simulink model "scdcascade_breach"  (R2020a)
settings: Solver=ode45  StartTime=0.0  StopTime=tspan(end)  RelTol=1e-3  EnableMultiTasking=on
PreLoadFcn:
  | Kp2 = 1.4817;
  | Ki2 = 4.7555;
  | Kp1 = 0.1575;
  | Ki1 = 0.042;
model workspace (MAT data in the model file):
  C1 = pidstd
  C1.IOSize_ = [1 1]
  C1.Data_ = ltipack.piddataS
  C1.Data_.Delay.Input = 0
  C1.Data_.Delay.Output = 0
  C1.Data_.Delay.IO = 0
  C1.Data_.Ts = 0
  C1.Data_.Kp = 0.1
  C1.Data_.Ti = 1
  C1.Data_.Td = 0
  C1.Data_.N = Inf
  C2 = pidstd
  C2.IOSize_ = [1 1]
  C2.Data_ = ltipack.piddataS
  C2.Data_.Delay.Input = 0
  C2.Data_.Delay.Output = 0
  C2.Data_.Delay.IO = 0
  C2.Data_.Ts = 0
  C2.Data_.Kp = 0.1
  C2.Data_.Ti = 1
  C2.Data_.Td = 0
  C2.Data_.N = Inf
  G1 = zpk
  G1.IOSize_ = [1 1]
  G1.Data_ = ltipack.zpkdata
  G1.Data_.z = {[]}
  G1.Data_.p = {[-1; -1; -1]}
  G1.Data_.k = 10
  G1.Data_.Delay.Input = 0
  G1.Data_.Delay.Output = 0
  G1.Data_.Delay.IO = 0
  G1.Data_.Ts = 0
  G2 = zpk
  G2.IOSize_ = [1 1]
  G2.Data_ = ltipack.zpkdata
  G2.Data_.z = {[]}
  G2.Data_.p = {-2}
  G2.Data_.k = 3
  G2.Data_.Delay.Input = 0
  G2.Data_.Delay.Output = 0
  G2.Data_.Delay.IO = 0
  G2.Data_.Ts = 0
libraries: cstblocks x2, simulink x1
settings Model: FPTRunName=Active  Creator=The MathWorks, Inc.  LastModifiedBy=nikhil
settings DataIOCC: ExternalInput=[t__, u__]  LoadExternalInput=on  SaveFormat=StructureWithTime
settings OptimizationCC: ExpressionDepthLimit=2147483647  LifeSpan=inf
settings DebuggingCC: UnderspecifiedInitializationDetection=Classic  MergeDetectMultiDrivingBlocksExec=none  SolverPrmCheckMsg=warning  FcnCallInpInsideContextMsg=warning  StateNameClashWarn=warning  SFUnexpectedBacktrackingDiag=warning  SFNoUnconditionalDefaultTransitionDiag=warning  SFExecutionAtInitializationDiag=none  ArithmeticOperatorsInVariantConditions=warning
settings HardwareCC: ProdBitPerPointer=32  ProdBitPerSizeT=32  ProdBitPerPtrDiffT=32  ProdLargestAtomicFloat=None  ProdIntDivRoundTo=Undefined  ProdEndianess=Unspecified  ProdWordSize=32  ProdHWDeviceType=32-bit Generic
settings ModelReferenceCC: PropagateSignalLabelsOutOfModel=off
settings SFSimCC: SimUseLocalCustomCode=off  CustomCodeUndefinedFunction=UseInterfaceOnly
settings RTWCC: RTWUseLocalCustomCode=off
settings CodeAppCC: StateflowObjectComments=on
settings GRTTargetCC: TargetLangStandard=C89/C90 (ANSI)  CombineOutputUpdateFcns=off  GRTInterface=on
settings ConfigComp: CovMetricSettings=dw  CovHtmlReporting=on  CovSaveCumulativeToWorkspaceVar=on  CovSaveSingleToWorkspaceVar=on  CovExternalEMLEnable=off  CovSFcnEnable=off

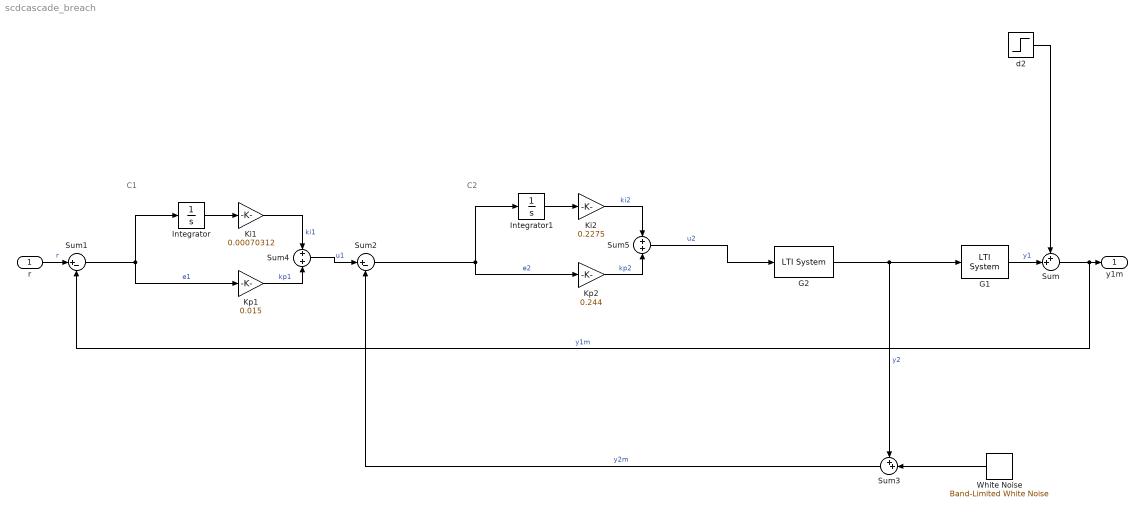
== system scdcascade_breach ==
  note: C2
  note: C1
  r : Inport
  G1 : cstblocks/LTI System  sys=G1  IC=[]
  G2 : cstblocks/LTI System  sys=G2  IC=[]
  Integrator : Integrator
  Integrator1 : Integrator
  Ki1 : Gain  Gain=0.00070312
  Ki2 : Gain  Gain=0.2275
  Kp1 : Gain  Gain=0.015
  Kp2 : Gain  Gain=0.244
  Sum : Sum  Inputs=++|
  Sum1 : Sum  Inputs=|+-
  Sum2 : Sum  Inputs=|+-
  Sum3 : Sum  Inputs=++|
  Sum4 : Sum
  Sum5 : Sum
  White Noise : simulink/Sources/Band-Limited White Noise  Cov=1e-5  Ts=0.1  seed=[23341]
  d2 : Step  Time=20  After=0.25  SampleTime=0
  y1m : Outport
  wires:
  G2/1 -> G1/1, Sum3/1  "y2"
  Sum5/1 -> G2/1  "u2"
  Sum2/1 -> Integrator1/1, Kp2/1  "e2"
  d2/1 -> Sum/1
  r/1 -> Sum1/1  "r"
  Sum1/1 -> Kp1/1, Integrator/1  "e1"
  Sum3/1 -> Sum2/2  "y2m"
  White Noise/1 -> Sum3/2
  G1/1 -> Sum/2  "y1"
  Sum/1 -> Sum1/2, y1m/1  "y1m"
  Sum4/1 -> Sum2/1  "u1"
  Ki1/1 -> Sum4/1  "ki1"
  Integrator/1 -> Ki1/1
  Kp1/1 -> Sum4/2  "kp1"
  Ki2/1 -> Sum5/1  "ki2"
  Integrator1/1 -> Ki2/1
  Kp2/1 -> Sum5/2  "kp2"
